simulink model "Project_Model"  (R2020b)
settings: Solver=VariableStepAuto  StartTime=0.0  StopTime=1.1  RelTol=1e-3
libraries: dspsrcs4 x5, slident x1, mpclib x1
settings Model: Creator=danie  LastModifiedBy=danie

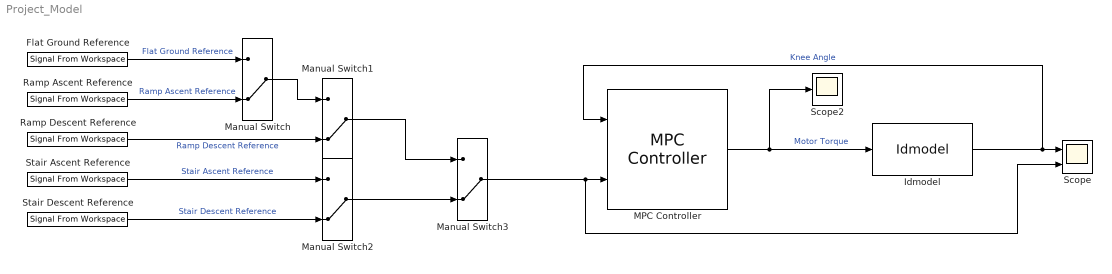
== system Project_Model ==
  Flat Ground Reference : dspsrcs4/Signal From Workspace  X=Flat_Ang_Ref  Ts=.01  nsamps=1  OutputAfterFinalValue=Setting to zero  ignoreOrWarnInputAndFrameLengths=off  OutputFrames=off
  Idmodel : slident/Models/Idmodel  sys=Knee_Torque_Plant  IC=0  noi=on  seed=[]
      settings: SourceProductBaseCode=ID
  MPC Controller : mpclib/MPC Controller  SCDEnableBlockLinearizationSpecification=on  mpcobj=mpc1  is_multiple=0  enable_value=0  return_u0=off  updateMPCinCallerWorkspace=on  md_inport=off  mv_inport=off  uref_inport=off  return_cost=off  return_mvseq=off  return_qpstatus=off  return_xseq=off  return_state=off  return_ovseq=off  state_inport=off  umin_inport=off  umax_inport=off  ymin_inport=off  ymax_inport=off  cc_inport=off  ywt_inport=off  uwt_inport=off  duwt_inport=off  rhoeps_inport=off  pm_inport=off  MaximumP=10  HorizonChoice=FixedHorizon  n_ts=0.01  n_p=8  n_mv=1  n_md=0  n_ud=0  n_mo=1  n_uo=0  BlockDataType=double  SampleTimeInherited=off  switch_inport=off
  Manual Switch{,1..3} (4 alike) : ManualSwitch  CurrentSetting=0
  Ramp Ascent Reference : dspsrcs4/Signal From Workspace  X=Ramp_Ascent_Ref  Ts=.01  nsamps=1  OutputAfterFinalValue=Setting to zero  ignoreOrWarnInputAndFrameLengths=off  OutputFrames=off
  Ramp Descent Reference : dspsrcs4/Signal From Workspace  X=Ramp_Descent_Ref  Ts=.01  nsamps=1  OutputAfterFinalValue=Setting to zero  ignoreOrWarnInputAndFrameLengths=off  OutputFrames=off
  Scope : Scope  NumInputPorts=2
  Scope2 : Scope
  Stair Ascent Reference : dspsrcs4/Signal From Workspace  X=Stair_Ascent_Ref  Ts=.01  nsamps=1  OutputAfterFinalValue=Setting to zero  ignoreOrWarnInputAndFrameLengths=off  OutputFrames=off
  Stair Descent Reference : dspsrcs4/Signal From Workspace  X=Stair_Descent_Ref  Ts=.01  nsamps=1  OutputAfterFinalValue=Setting to zero  ignoreOrWarnInputAndFrameLengths=off  OutputFrames=off
  wires:
  Idmodel/1 -> MPC Controller/1, Scope/1  "Knee Angle"
  MPC Controller/1 -> Scope2/1, Idmodel/1  "Motor Torque"
  Manual Switch3/1 -> Scope/2, MPC Controller/2
  Flat Ground Reference/1 -> Manual Switch/1  "Flat Ground Reference"
  Ramp Ascent Reference/1 -> Manual Switch/2  "Ramp Ascent Reference"
  Ramp Descent Reference/1 -> Manual Switch1/2  "Ramp Descent Reference"
  Stair Ascent Reference/1 -> Manual Switch2/1  "Stair Ascent Reference"
  Stair Descent Reference/1 -> Manual Switch2/2  "Stair Descent Reference"
  Manual Switch/1 -> Manual Switch1/1
  Manual Switch2/1 -> Manual Switch3/2
  Manual Switch1/1 -> Manual Switch3/1
